simulink model "Ej1"  (R2018a)
settings: Solver=VariableStepAuto  StartTime=0.0  StopTime=100  RelTol=1e-3
values from neighbouring files (symbols this model uses):
  a = 200    [Ej1_params.m]    (also in Ej2_params.m; Ej3_params.m; Ej4_params.m)
  b = 10000    [Ej1_params.m]    (also in Ej2_params.m; Ej3_params.m; Ej4_params.m)
  g = 9.82    [Ej1_params.m]    (also in Ej2_params.m; Ej3_params.m; Ej4_params.m)
  G_c = .01 * (30 / 12.43) * (30 /33.6)    (= 0.021549247213)    [Ej1_params.m]    (also in Ej2_params.m = 1; Ej5_G_c.m = zpk([-1/a -1/b], 0, K*a*b); Ej8_G_c.m = G_c / A; G_c_Ej5.m = zpk([-1/a -1/b], 0, K*a*b))
  m = 1500    [Ej1_params.m]    (also in Ej2_params.m = 1000; Ej3_params.m = 1000; Ej4_params.m = 1000)
settings Model: Creator=joses  LastModifiedBy=joses

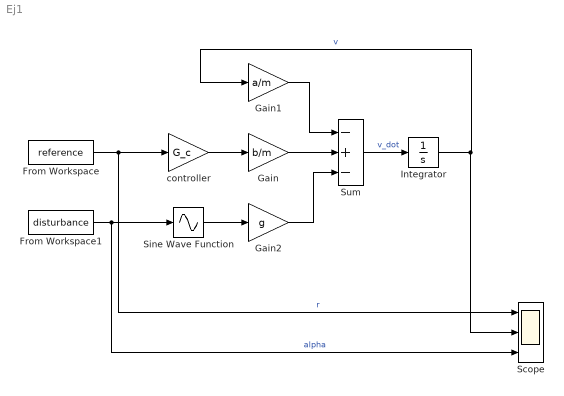
== system Ej1 ==
  From Workspace : FromWorkspace  VariableName=reference  SampleTime=.01
  From Workspace1 : FromWorkspace  VariableName=disturbance  SampleTime=.01
  Gain : Gain  Gain=b/m
  Gain1 : Gain  Gain=a/m
  Gain2 : Gain  Gain=g
  Integrator : Integrator
  Scope : Scope  NumInputPorts=3
  Sine Wave Function : Sin  TimeSource=Use external signal  SampleTime=0
  Sum : Sum  Inputs=-+-
  controller : Gain  Gain=G_c
  wires:
  Sum/1 -> Integrator/1  "v_dot"
  Gain/1 -> Sum/2
  Gain1/1 -> Sum/1
  Integrator/1 -> Scope/2, Gain1/1  "v"
  controller/1 -> Gain/1
  From Workspace/1 -> controller/1, Scope/1  "r"
  Sine Wave Function/1 -> Gain2/1
  From Workspace1/1 -> Scope/3, Sine Wave Function/1  "alpha"
  Gain2/1 -> Sum/3
